simulink model "LCK_AVP"  (R2018b)
settings: Solver=FixedStepDiscrete  StartTime=0.0  StopTime=inf  FixedStep=0.01  RelTol=1e-3
PreLoadFcn:
  | if exist('tl_preloadfcn','file'), tl_preloadfcn(gcs,'4.4.0.41'); end
PostLoadFcn:
  | if any(exist('dsrtsu_mdlpostloadfcn', 'file') ~= 0), dsrtsu_mdlpostloadfcn('Execute', bdroot); end
  | if exist('tl_postloadfcn','file'), tl_postloadfcn(gcs,'4.4.0.41'); end
InitFcn:
  | if exist('tlds_init','file'), tlds_init(gcs); end
StartFcn:
  | if exist('tlds_start','file'), tlds_start(gcs); end
StopFcn:
  | if exist('tlds_stop','file'), tlds_stop(gcs); end
values from neighbouring files (symbols this model uses):
  C_DEG2RAD = 0.0175    [LCK_Macro.sldd]
  C_KPH2MPS = 0.2778    [LCK_Macro.sldd]
  C_NEARZERO = 0.0001    [LCK_Macro.sldd]
  C_ONE = 1.0    [LCK_Macro.sldd]
  C_RAD2DEG = 57.2958    [LCK_Macro.sldd]
  C_ZERO = 0.0    [LCK_Macro.sldd]
  k_accel_pedal_pos_per_speed_x : value not decoded    [LCK_LogicPara.sldd]
  k_accel_pedal_pos_per_speed_z : value not decoded    [LCK_LogicPara.sldd]
  k_brake_suprress_hold = 1000.0    [LCK_LogicPara.sldd]
  k_driver_appl_torque_filt = 50.0    [LCK_LogicPara.sldd]
  k_driver_suppression_hold_time = 3000.0    [LCK_LogicPara.sldd]
  k_hands_on_wheel_hold_msec = 500.0    [LCK_LogicPara.sldd]
  k_hands_on_wheel_torque_hi = 0.2    [LCK_LogicPara.sldd]
  k_hands_on_wheel_torque_lo = 0.15    [LCK_LogicPara.sldd]
  k_handsoff_delay_cycles = 50.0    [LCK_LogicPara.sldd]
  k_handsoff_torq_Lo_CR = 0.3    [LCK_LogicPara.sldd]
  k_handson_delay_cycles = 5.0    [LCK_LogicPara.sldd]
  k_HighAccel_suppress_hold = 3000.0    [LCK_LogicPara.sldd]
  k_HLR_suprress_hold = 3000.0    [LCK_LogicPara.sldd]
  k_hs_StrAng_CR_threshold_z : value not decoded    [LCK_LogicPara.sldd]
  k_LC_Exit_Switch = 0.0    [LCK_LogicPara.sldd]
  k_LCG_Configured = 1.0    [LCK_LogicPara.sldd]
  k_LCK_A0_Rdy2Act_UseConst = 0.0    [LCK_LogicPara.sldd]
  k_LCK_A0Fac_ActSta : value not decoded    [LCK_CtrlPara.sldd]
  k_LCK_A0Fac_DrvStm : value not decoded    [LCK_CtrlPara.sldd]
  k_LCK_A0Shift_LftCurv : value not decoded    [LCK_CtrlPara.sldd]
  k_LCK_A0Shift_RgtCurv : value not decoded    [LCK_CtrlPara.sldd]
  k_LCK_A0Shift_StraLan = 0.0    [LCK_CtrlPara.sldd]
  k_LCK_A0ShiftFac_Dy_LftCurv : value not decoded    [LCK_CtrlPara.sldd]
  k_LCK_A0ShiftFac_Dy_RgtCurv : value not decoded    [LCK_CtrlPara.sldd]
  k_LCK_A0ShiftFac_Vspd : value not decoded    [LCK_CtrlPara.sldd]
  k_LCK_accel_inhibit_thold = 35.0    [LCK_LogicPara.sldd]
  k_LCK_Active2Ready_Mask = 255.0    [LCK_LogicPara.sldd]
  k_LCK_CvatRateBks : value not decoded    [LCK_CtrlPara.sldd]
  k_LCK_CvatrBks : value not decoded    [LCK_CtrlPara.sldd]
  k_LCK_DFac_Dy : value not decoded    [LCK_CtrlPara.sldd]
  k_LCK_DFac_Dy_Curv : value not decoded    [LCK_CtrlPara.sldd]
  k_LCK_DFac_HaCurCen : value not decoded    [LCK_CtrlPara.sldd]
  k_LCK_DFac_HaCurSid : value not decoded    [LCK_CtrlPara.sldd]
  k_LCK_DFac_HadCurCen : value not decoded    [LCK_CtrlPara.sldd]
  k_LCK_DFac_HadCurSid : value not decoded    [LCK_CtrlPara.sldd]
  k_LCK_DFac_HadStrCen : value not decoded    [LCK_CtrlPara.sldd]
  k_LCK_DFac_HadStrSid : value not decoded    [LCK_CtrlPara.sldd]
  k_LCK_DFac_HaStrCen : value not decoded    [LCK_CtrlPara.sldd]
  k_LCK_DFac_HaStrSid : value not decoded    [LCK_CtrlPara.sldd]
  k_LCK_DFac_Rad : value not decoded    [LCK_CtrlPara.sldd]
  k_LCK_DFac_SA_CurCen : value not decoded    [LCK_CtrlPara.sldd]
  k_LCK_DFac_SA_CurSid : value not decoded    [LCK_CtrlPara.sldd]
  k_LCK_DFac_SA_StrCen : value not decoded    [LCK_CtrlPara.sldd]
  k_LCK_DFac_SA_StrSid : value not decoded    [LCK_CtrlPara.sldd]
  k_LCK_DFac_SS_CurCen : value not decoded    [LCK_CtrlPara.sldd]
  k_LCK_DFac_SS_CurSid : value not decoded    [LCK_CtrlPara.sldd]
  k_LCK_DFac_SS_StrCen : value not decoded    [LCK_CtrlPara.sldd]
  k_LCK_DFac_SS_StrSid : value not decoded    [LCK_CtrlPara.sldd]
  k_LCK_DFac_Vspd : value not decoded    [LCK_CtrlPara.sldd]
  k_LCK_DlyTm_DrvStim = 0.2    [LCK_CtrlPara.sldd]
  k_LCK_DTermMax = 2.0    [LCK_CtrlPara.sldd]
  k_LCK_DyBks_Curv : value not decoded    [LCK_CtrlPara.sldd]
  k_LCK_Enable_POOnly = 1.0    [LCK_LogicPara.sldd]
  k_LCK_Entry_DistBuffer = 0.1    [LCK_LogicPara.sldd]
  k_LCK_Fac_Vspd2RngThr_FalRec = 0.23    [LCK_CtrlPara.sldd]
  k_LCK_Ffw_CvatSwh = 0.0    [LCK_CtrlPara.sldd]
  k_LCK_Ffw_DyBks : value not decoded    [LCK_CtrlPara.sldd]
  k_LCK_Ffw_TimCon_CmdFlt = 0.0    [LCK_CtrlPara.sldd]
  k_LCK_FfwDeltaFac_Rad_Lft : value not decoded    [LCK_CtrlPara.sldd]
  k_LCK_FfwDeltaFac_Rad_Rgt : value not decoded    [LCK_CtrlPara.sldd]
  k_LCK_FfwDeltaFac_Vspd : value not decoded    [LCK_CtrlPara.sldd]
  k_LCK_FfwFac_CvatRate_Lft : value not decoded    [LCK_CtrlPara.sldd]
  k_LCK_FfwFac_CvatRate_Rgt : value not decoded    [LCK_CtrlPara.sldd]
  k_LCK_FfwFac_Dy : value not decoded    [LCK_CtrlPara.sldd]
  k_LCK_FfwFac_Rad_Lft : value not decoded    [LCK_CtrlPara.sldd]
  k_LCK_FfwFac_Rad_Rgt : value not decoded    [LCK_CtrlPara.sldd]
  k_LCK_FfwFac_Vspd : value not decoded    [LCK_CtrlPara.sldd]
  k_LCK_FfwTorq_Cvat : value not decoded    [LCK_CtrlPara.sldd]
  k_LCK_HAFac_ActSta : value not decoded    [LCK_CtrlPara.sldd]
  k_LCK_HAFac_DrvStm : value not decoded    [LCK_CtrlPara.sldd]
  k_LCK_HaloTime = 2000.0    [LCK_LogicPara.sldd]
  k_LCK_HaloTime_Switch = 0.0    [LCK_LogicPara.sldd]
  k_LCK_HARFac_ActSta : value not decoded    [LCK_CtrlPara.sldd]
  k_LCK_HARFac_DrvStm : value not decoded    [LCK_CtrlPara.sldd]
  k_LCK_Hed_DyBks : value not decoded    [LCK_CtrlPara.sldd]
  k_LCK_HedAngDiffX : value not decoded    [LCK_CtrlPara.sldd]
  k_LCK_HedAngRateDiffX : value not decoded    [LCK_CtrlPara.sldd]
  k_LCK_HndsOnWhel_DlyTm_Idl2Rdy = 0.0    [LCK_LogicPara.sldd]
  k_LCK_host_veh_width = 1.86    [LCK_LogicPara.sldd]
  k_LCK_Idle2Ready_Mask = 239.0    [LCK_LogicPara.sldd]
  k_LCK_Junc_SusTime = 1.0    [LCK_LogicPara.sldd]
  k_LCK_KpKdDecSlopeLmt = 10.0    [LCK_CtrlPara.sldd]
  k_LCK_KpKdIncSlopeLmt = 5.0    [LCK_CtrlPara.sldd]
  k_LCK_Lat_Ctrl_DFac_Lft = 1.0    [LCK_CtrlPara.sldd]
  k_LCK_Lat_Ctrl_DFac_Rgt = 1.05    [LCK_CtrlPara.sldd]
  k_LCK_Lat_Ctrl_Kd = 0.8    [LCK_CtrlPara.sldd]
  k_LCK_Lat_Ctrl_Ki = 0.5    [LCK_CtrlPara.sldd]
  k_LCK_Lat_Ctrl_Kp = 0.7    [LCK_CtrlPara.sldd]
  k_LCK_Lat_Ctrl_Kp_NearGain = 0.7    [LCK_CtrlPara.sldd]
  k_LCK_Lat_Ctrl_PFac_Lft = 1.0    [LCK_CtrlPara.sldd]
  k_LCK_Lat_Ctrl_PFac_Rgt = 1.05    [LCK_CtrlPara.sldd]
  k_LCK_Lat_Ctrl_TimCon_CmdFlt = 5.0    [LCK_CtrlPara.sldd]
  k_LCK_Lat_DFac_Rad : value not decoded    [LCK_CtrlPara.sldd]
  k_LCK_Lat_DFac_SS_Cur : value not decoded    [LCK_CtrlPara.sldd]
  k_LCK_Lat_DFac_SS_Str : value not decoded    [LCK_CtrlPara.sldd]
  k_LCK_Lat_DFac_Vspd : value not decoded    [LCK_CtrlPara.sldd]
  k_LCK_Lat_DyBks : value not decoded    [LCK_CtrlPara.sldd]
  k_LCK_Lat_IFac_Rad : value not decoded    [LCK_CtrlPara.sldd]
  k_LCK_Lat_IFac_Vspd : value not decoded    [LCK_CtrlPara.sldd]
  k_LCK_Lat_ILmtFac_Dy_CurvLan : value not decoded    [LCK_CtrlPara.sldd]
  k_LCK_Lat_ILmtFac_Dy_StraLan : value not decoded    [LCK_CtrlPara.sldd]
  k_LCK_Lat_ILmtFac_Rad : value not decoded    [LCK_CtrlPara.sldd]
  k_LCK_Lat_ILmtFac_Rad_NearGain = 1.0    [LCK_CtrlPara.sldd]
  k_LCK_Lat_ILmtFac_Vspd_CurvLan : value not decoded    [LCK_CtrlPara.sldd]
  k_LCK_Lat_ILmtFac_Vspd_StraLan : value not decoded    [LCK_CtrlPara.sldd]
  k_LCK_Lat_ITermLmt_Dy = 1.0    [LCK_CtrlPara.sldd]
  k_LCK_Lat_KpKdDecSlopeLmt = 10.0    [LCK_CtrlPara.sldd]
  k_LCK_Lat_KpKdIncSlopeLmt = 10.0    [LCK_CtrlPara.sldd]
  k_LCK_Lat_PFac_Dy_InnLftCur : value not decoded    [LCK_CtrlPara.sldd]
  k_LCK_Lat_PFac_Dy_InnRgtCur : value not decoded    [LCK_CtrlPara.sldd]
  k_LCK_Lat_PFac_Dy_OutLftCur : value not decoded    [LCK_CtrlPara.sldd]
  k_LCK_Lat_PFac_Dy_OutRgtCur : value not decoded    [LCK_CtrlPara.sldd]
  k_LCK_Lat_PFac_Dy_Str : value not decoded    [LCK_CtrlPara.sldd]
  k_LCK_Lat_PFac_Rad : value not decoded    [LCK_CtrlPara.sldd]
  ... (+153 more)
undefined symbols (not defined in the file or in its folder): k_LCK_CurvBks, K_LCK_SPA0A1A2_LMRngCmp_y
libraries: LateralControl_fcns_lib x58, simulink x24
(part 3 of 48)

== system LCK_AVP/Lateral_Control_Module/LCK_State_Ctrl ==
  LatCtrl_LCK_LanSigInputs : Inport  Description=_GWMAB30P4.LCK.000_87_  OutDataTypeStr=Bus: LatCtrl_LCK_LanSigInputs_t
  LatCtrl_LCK_VehSigInputs : Inport  Description=_GWMAB30P4.LCK.000_287_  Port=2  OutDataTypeStr=Bus: LatCtrl_LCK_VehSigInputs_t
  LatCtrl_LCK_SPPInfo : Inport  Description=_GWMAB30P4.LCK.000_87_  Port=3  OutDataTypeStr=Bus: LatCtrl_LCK_SPPInfo_t
  Final_Torq_Cmd : Inport  Port=4
  LC_Info : Inport  Port=5
  TJA_State : Inport  Description=_GWMAB30P4.LCK.000_80_  Port=6
  ZOP_LCK_Activate : Inport  Description=_GWMAB30P4.LCK.000_80_  Port=7
  ZOP_LC_Command : Inport  Port=8
  PO_Enable : Inport  Port=9
  Bus Creator : BusCreator  Inputs=5
  Bus Creator1 : BusCreator  Inputs=5
  Bus Selector : BusSelector  OutputSignals=Vehicle_Speed,Steer_Torq,Steer_Ang,BrkPedalApplied,AccPedalPosition,Gear_Pos,Steer_Spd,DirectionIndSwitchPos
  Bus Selector1 : BusSelector  OutputSignals=Vehicle_Speed,LDWLKASwReq
  Bus Selector2 : BusSelector  OutputSignals=Veh_Yaw_Rate,LKATrqOvrlTrqDStat,DirectionIndSwitchPos
  Bus Selector3 : BusSelector  OutputSignals=VID_Lane_Width,VID_Lin_01_Range,VID_Lin_02_Range,VID_Lin_01_Type,VID_Lin_02_Type
  Bus Selector4 : BusSelector  OutputSignals=SPP_Conf,SPP_Type,SPP_A0,SPP_A1,SPP_A2
  Bus Selector5 : BusSelector  OutputSignals=LC_Phase
  Constant1 : Constant  Tag={'output',{'type','Int32'},'date',737184.60397266201}  Description=_GWMAB30P2.LCK.000_1069_  Value=0
  Constant3 : Constant  Tag={'output',{'type','Int32'},'date',737184.60397266201}  Description=_GWMAB30P2.LCK.000_1069_  Value=0
  Data Type Conversion{,1..3} (4 alike) : DataTypeConversion  OutDataTypeStr=single
  Det_Driver_Operation : Subsystem
  Gain : Gain
  LCK Mode Manager : Stateflow chart  TreatAsAtomicUnit=on
  LCK_Mode_Transition : Subsystem
  LCK_Mode : Outport  Description=_GWMAB30P4.LCK.000_194_
  LCK_State_Info : Outport  Description=_GWMAB30P4.LCK.000_194_  Port=2
  Driver_Operation_Info : Outport  Description=_GWMAB30P4.LCK.000_194_  Port=3
  wires:
  LCK_Mode_Transition/21(READY2ACTIVE_Magic_Out) -> Data Type Conversion2/1  "READY2ACTIVE_Magic_Out"
  LCK_Mode_Transition/22(ACTIVE2READY_Magic_Out) -> Data Type Conversion3/1  "ACTIVE2READY_Magic_Out"
  Bus Creator/1 -> LCK_State_Info/1
  LCK_Mode_Transition/5(READY2OFF) -> LCK Mode Manager/5(READY2OFF)
  LCK_Mode_Transition/8(ACTIVE2OFF) -> LCK Mode Manager/8(ACTIVE2OFF)
  LCK_Mode_Transition/11(ERROR2OFF) -> LCK Mode Manager/11(ERROR2OFF)
  LCK_Mode_Transition/4(IDLE2READY) -> LCK Mode Manager/4(IDLE2READY)
  LCK_Mode_Transition/2(OFF2READY) -> LCK Mode Manager/2(OFF2READY)
  LCK_Mode_Transition/1(OFF2IDLE) -> LCK Mode Manager/1(OFF2IDLE)
  LCK_Mode_Transition/3(IDLE2OFF) -> LCK Mode Manager/3(IDLE2OFF)
  LCK_Mode_Transition/7(READY2ACTIVE) -> LCK Mode Manager/7(READY2ACTIVE)
  LCK_Mode_Transition/6(READY2IDLE) -> LCK Mode Manager/6(READY2IDLE)
  LCK_Mode_Transition/9(ACTIVE2IDLE) -> LCK Mode Manager/9(ACTIVE2IDLE)
  LCK_Mode_Transition/19(IDLE2READY_Magic_Out) -> Data Type Conversion/1  "IDLE2READY_Magic_Out"
  LCK_Mode_Transition/20(READY2IDLE_Magic_Out) -> Data Type Conversion1/1  "READY2IDLE_Magic_Out"
  LCK_Mode_Transition/13(ERROR2READY) -> LCK Mode Manager/13(ERROR2READY)
  LCK_Mode_Transition/12(ERROR2IDLE) -> LCK Mode Manager/12(ERROR2IDLE)
  LCK_Mode_Transition/10(ACTIVE2READY) -> LCK Mode Manager/10(ACTIVE2READY)
  LCK_Mode_Transition/14(ERROR_CONDITION) -> LCK Mode Manager/14(ERROR_CONDITION)
  Det_Driver_Operation/5(f_Right_driver_suppression) -> Bus Creator1/5, LCK_Mode_Transition/23(f_right_driver_suppression)
  Det_Driver_Operation/1(f_hands_on_wheel) -> Bus Creator1/1, LCK_Mode_Transition/19(f_hands_on_wheel)  "f_hands_on_wheel"
  Det_Driver_Operation/2(f_driver_override_left_trq) -> Bus Creator1/2, LCK_Mode_Transition/20(f_driv_override_left)
  Bus Selector2/1 -> LCK_Mode_Transition/13(yaw_deg_iso_filt)  "<Veh_Yaw_Rate>"
  Bus Selector2/2 -> LCK_Mode_Transition/14(LKATrqOvrlTrqDStat)  "<LKATrqOvrlTrqDStat>"
  [LCK_Mode] -> LCK_Mode_Transition/16(LCK_Mode)
  Constant3/1 -> LCK_Mode_Transition/17(LeftLaneChange)
  Constant1/1 -> LCK_Mode_Transition/18(RightLaneChange)
  Bus Selector/2 -> Det_Driver_Operation/2(TorsionBarTorque)  "<Steer_Torq>"
  [LCK_Mode] -> Det_Driver_Operation/9(LCK_Mode)
  Final_Torq_Cmd/1 -> Det_Driver_Operation/10(Final_Torq_Cmd)
  Bus Selector/7 -> Det_Driver_Operation/7(steer_angle_CR_iso)  "<Steer_Spd>"
  Bus Selector/4 -> Det_Driver_Operation/4(BrkPedalApp)  "<BrkPedalApplied>"
  Bus Selector/3 -> Det_Driver_Operation/3(Steer_Angle_iso)  "<Steer_Ang>"
  Bus Selector/5 -> Det_Driver_Operation/5(AccPedalPosition)  "<AccPedalPosition>"
  Bus Selector/6 -> Det_Driver_Operation/6(Gear_Pos)  "<Gear_Pos>"
  Bus Selector/1 -> Det_Driver_Operation/1(veh_speed_kph)  "<Vehicle_Speed>"
  LatCtrl_LCK_VehSigInputs/1 -> [LatCtrl_LCK_VehSigInputs], Bus Selector/1
  [LatCtrl_LCK_VehSigInputs] -> Bus Selector1/1
  Bus Selector1/2 -> LCK_Mode_Transition/2(LDWLKASwReq)  "<LDWLKASwReq>"
  Bus Selector1/1 -> LCK_Mode_Transition/1(Veh_Speed_kph)  "<Vehicle_Speed>"
  [LatCtrl_LCK_VehSigInputs] -> Bus Selector2/1
  [LCK_Mode] -> Bus Creator/5
  Bus Selector/8 -> Det_Driver_Operation/8(DirectionIndSwitchPos)  "<DirectionIndSwitchPos>"
  Bus Selector3/1 -> LCK_Mode_Transition/8(curr_lane_width)  "<VID_Lane_Width>"
  Bus Selector3/2 -> LCK_Mode_Transition/9(VIS_LANE_LEFT_INDIVID_RANGE)  "<VID_Lin_01_Range>"
  Bus Selector3/3 -> LCK_Mode_Transition/10(VIS_LANE_RIGHT_INDIVID_RANGE)  "<VID_Lin_02_Range>"
  LatCtrl_LCK_LanSigInputs/1 -> Bus Selector3/1
  LatCtrl_LCK_SPPInfo/1 -> Bus Selector4/1
  Bus Selector4/3 -> LCK_Mode_Transition/5(SPP_A0)  "<SPP_A0>"
  Bus Selector4/4 -> LCK_Mode_Transition/6(SPP_A1)  "<SPP_A1>"
  Bus Selector4/5 -> LCK_Mode_Transition/7(SPP_A2)  "<SPP_A2>"
  Data Type Conversion/1 -> Bus Creator/1
  Data Type Conversion1/1 -> Bus Creator/2
  Data Type Conversion2/1 -> Bus Creator/3
  Data Type Conversion3/1 -> Bus Creator/4
  Gain/1 -> [LCK_Mode]
  Bus Creator1/1 -> Driver_Operation_Info/1
  Bus Selector4/1 -> LCK_Mode_Transition/3(SP_conf)  "<SPP_Conf>"
  Bus Selector4/2 -> LCK_Mode_Transition/4(SP_type)  "<SPP_Type>"
  LCK_Mode_Transition/15(LCK2LEFTLC) -> LCK Mode Manager/15(LCK2LEFTLC)
  LCK_Mode_Transition/16(LCK2RIGHTLC) -> LCK Mode Manager/16(LCK2RIGHTLC)
  LCK_Mode_Transition/17(LEFTLC2LCK) -> LCK Mode Manager/17(LEFTLC2LCK)
  LCK_Mode_Transition/18(RIGHTLC2LCK) -> LCK Mode Manager/18(RIGHTLC2LCK)
  LCK Mode Manager/1(LCK_Mode) -> Gain/1, LCK_Mode/1  "LCK_Mode"
  LC_Info/1 -> Bus Selector5/1
  Bus Selector5/1 -> LCK_Mode_Transition/24(LC_Phase)  "<LC_Phase>"
  Det_Driver_Operation/3(f_driver_override_right_trq) -> Bus Creator1/3, LCK_Mode_Transition/21(f_driv_override_right)
  Det_Driver_Operation/4(f_Left_driver_suppression) -> Bus Creator1/4, LCK_Mode_Transition/22(f_left_driver_suppression)
  Bus Selector2/3 -> LCK_Mode_Transition/15(DirectionIndSwitchPos)  "<DirectionIndSwitchPos>"
  ZOP_LC_Command/1 -> LCK_Mode_Transition/27(ZOP_LC_Command)
  ZOP_LCK_Activate/1 -> LCK_Mode_Transition/26(ZOP_LCK_Activate)
  TJA_State/1 -> LCK_Mode_Transition/25(TJA_State)
  Bus Selector3/4 -> LCK_Mode_Transition/11(Lin01_Type)  "<VID_Lin_01_Type>"
  Bus Selector3/5 -> LCK_Mode_Transition/12(Lin02_Type)  "<VID_Lin_02_Type>"
  PO_Enable/1 -> LCK_Mode_Transition/28(PO_Enable)
